simulink model "HT_dk_theo_mo_hinh_chuan"  (R2023a)
settings: Solver=ode4  StartTime=0.0  StopTime=50  FixedStep=0.001  RelTol=1e-3
settings Model: Creator=VINH  LastModifiedBy=VINH

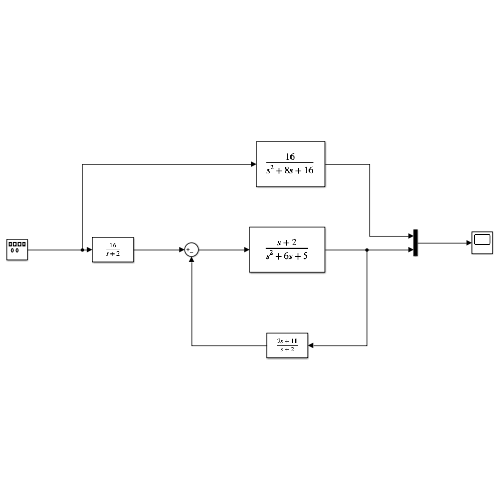
[thumbnail: Simulink's stored preview of the top-level diagram]
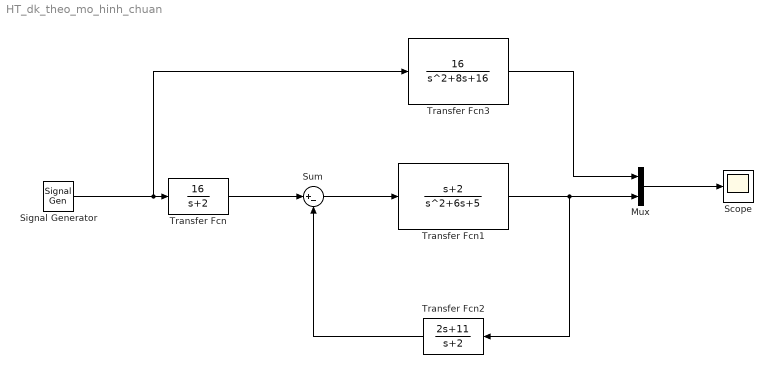
== system HT_dk_theo_mo_hinh_chuan ==
  Mux : Mux  Inputs=2
  Scope : Scope
  Signal Generator : SignalGenerator  WaveForm=square  Amplitude=0.5  Frequency=0.1
  Sum : Sum  Inputs=|+-
  Transfer Fcn : TransferFcn  Numerator=[16]  Denominator=[1 2]
  Transfer Fcn1 : TransferFcn  Numerator=[1 2]  Denominator=[1 6 5]
  Transfer Fcn2 : TransferFcn  Numerator=[2 11]  Denominator=[1 2]
  Transfer Fcn3 : TransferFcn  Numerator=[16]  Denominator=[1 8 16]
  wires:
  Transfer Fcn/1 -> Sum/1
  Signal Generator/1 -> Transfer Fcn3/1, Transfer Fcn/1
  Sum/1 -> Transfer Fcn1/1
  Transfer Fcn1/1 -> Transfer Fcn2/1, Mux/2
  Transfer Fcn2/1 -> Sum/2
  Transfer Fcn3/1 -> Mux/1
  Mux/1 -> Scope/1
